simulink model "Open_scen_lucie_test_cs"  (R2019a)
settings: Solver=ode5  StartTime=0.0  StopTime=60  FixedStep=1/60  RelTol=1e-3
PreLoadFcn:
  | mbxruntime.callbacks.PreLoadFcn(bdroot);
PostLoadFcn:
  | mbxruntime.callbacks.PostLoadFcn(bdroot);
InitFcn:
  | mbxruntime.callbacks.InitFcn(bdroot);
StartFcn:
  | mbxruntime.callbacks.StartFcn(bdroot);
StopFcn:
  | mbxruntime.callbacks.StopFcn(bdroot);
model workspace: external: MAT-File .\Open_scen_lucie_test_cs_hws.mat (data not in the file)
undefined symbols (not defined in the file or in its folder): DiscIntNeverNeededParam, FovAzimuth, FovAzimuthDefined, FovElevation, FovElevationDefined, InitImageOutputDir, LocationX, LocationXDefined, LocationY, LocationYDefined, LocationZ, LocationZDefined, mbxruntime, Open_scen_lucie_test_cs_05b3fdca6ec99adc, Open_scen_lucie_test_cs_2d1bc0fbf6141b87, Open_scen_lucie_test_cs_453760b7ad36561d, Open_scen_lucie_test_cs_54de7300b247ce0d, Open_scen_lucie_test_cs_6819f386244a4b71, Open_scen_lucie_test_cs_685351e056f1bd0b, Open_scen_lucie_test_cs_6cd7f038842b0b77, Open_scen_lucie_test_cs_7a35ff65ce771bf6, Open_scen_lucie_test_cs_7ca083c9065fb1a1, Open_scen_lucie_test_cs_8bffacb258fa391b, Open_scen_lucie_test_cs_90e3bd399387ee5e, Open_scen_lucie_test_cs_a1176fb0c2e52fd1, Open_scen_lucie_test_cs_bb93306955583605, Open_scen_lucie_test_cs_c100ca66a180e443, Open_scen_lucie_test_cs_c1ddb1ec4c47a5f8, Open_scen_lucie_test_cs_ee3cfcef3d4d50fa, Open_scen_lucie_test_cs_f0142b471b498fb5, Open_scen_lucie_test_cs_fad1968c5de81336, OrientationPitch, OrientationPitchDefined, OrientationRoll, OrientationRollDefined, OrientationYaw, OrientationYawDefined, tabledata
libraries: adeye_lib x15, PreScanSimulinkLibrary x6, PreScanUsefulBlocks x1, simulink x1
(part 2 of 8)

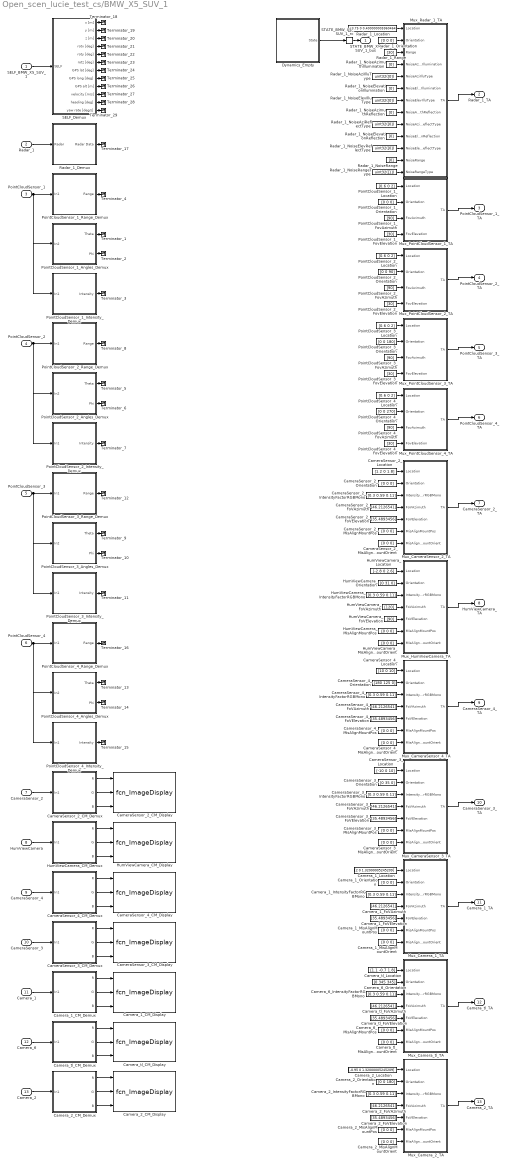
== system Open_scen_lucie_test_cs/BMW_X5_SUV_1 ==
  SELF_BMW_X5_SUV_1 : Inport  Tag=inport/SelfPort  OutDataTypeStr=Bus: PRESCAN_SELFSENSORDATA  PortDimensions=1  SampleTime=1/60  BusOutputAsStruct=on
  Radar_1 : Inport  Tag=inport/Radar  Port=2  OutDataTypeStr=Bus: PRESCAN_SCANNERSENSOR_MESSAGE  PortDimensions=7  SampleTime=1/20  BusOutputAsStruct=on
  PointCloudSensor_1 : Inport  Tag=inport/PointCloudInport  Port=3  OutDataTypeStr=single  SampleTime=1/20  BusOutputAsStruct=on
  PointCloudSensor_2 : Inport  Tag=inport/PointCloudInport  Port=4  OutDataTypeStr=single  SampleTime=1/20  BusOutputAsStruct=on
  PointCloudSensor_3 : Inport  Tag=inport/PointCloudInport  Port=5  OutDataTypeStr=single  SampleTime=1/20  BusOutputAsStruct=on
  PointCloudSensor_4 : Inport  Tag=inport/PointCloudInport  Port=6  OutDataTypeStr=single  SampleTime=1/20  BusOutputAsStruct=on
  CameraSensor_2 : Inport  Tag=inport/Camera/CameraSensor  Port=7  OutDataTypeStr=uint8  SampleTime=1/20  BusOutputAsStruct=on
  HumViewCamera : Inport  Tag=inport/Camera/CameraSensor  Port=8  OutDataTypeStr=uint8  SampleTime=1/60  BusOutputAsStruct=on
  CameraSensor_4 : Inport  Tag=inport/Camera/CameraSensor  Port=9  OutDataTypeStr=uint8  SampleTime=1/20  BusOutputAsStruct=on
  CameraSensor_3 : Inport  Tag=inport/Camera/CameraSensor  Port=10  OutDataTypeStr=uint8  SampleTime=1/20  BusOutputAsStruct=on
  Camera_1 : Inport  Tag=inport/Camera/CameraSensor  Port=11  OutDataTypeStr=uint8  SampleTime=1/20  BusOutputAsStruct=on
  Camera_tl : Inport  Tag=inport/Camera/CameraSensor  Port=12  OutDataTypeStr=uint8  SampleTime=1/20  BusOutputAsStruct=on
  Camera_2 : Inport  Tag=inport/Camera/CameraSensor  Port=13  OutDataTypeStr=uint8  SampleTime=1/20  BusOutputAsStruct=on
  CameraSensor_2_CM_Demux : Subsystem  Tag=demux/Camera/Color  mask{SensorName=CameraSensor_2, hres=960, vres=720}
      mask prompts: SensorName "Sensor Name"; hres "Horizontal Resolution"; vres "Vertical Resolution"
      mask Help: eval('openHelp(457)')
      mask Display:
      | fprintf('MONO CAMERA:\n Color\n %s \n %d x %d px',SensorName,hres,vres)
      | port_label('output',1,'R')
      | port_label('output',2,'G')
      | port_label('output',3,'B')
  CameraSensor_2_CM_Display : M-S-Function  Tag=CameraSensor_Color_Display  InitFcn=InitImageOutputDir(gcb);  FunctionName=fcn_ImageDisplay  Parameters=SensorName EnableDisplay EnablePosition DisplayPosition FigureHandle SaveResults BitmapFormat TempOutputDir CameraType DataType  mask(PreScan Color Display Block){SensorName=CameraSensor_2, EnableDisplay=on, EnablePosition=off, DisplayPosition=[10 10 960 720], FigureHandle=40605, SaveResults=off, Format=PNG, TempOutputDir=0, CameraType=Mono, DataType=uint8}
      mask prompts: SensorName "User Specified: Title of Display"; EnableDisplay "Active"; EnablePosition "Set Display window position"; DisplayPosition "Display window position [xpos ypos width height]"; FigureHandle "Unique Handle"; SaveResults "Save results"; TempOutputDir "OutputDir"; CameraType "Camera Type"; DataType "Image Data Type"
      mask help: This block displays the RGB output of a PreScan camera sensor.
      mask init:
      | if EnableDisplay
      |     EnableString='';
      |     EnableColor='gray';
      | else
      |     EnableString='INACTIVE';
      |     EnableColor='red';
      | end
      | switch Format
      |     case 1
      |         BitmapFormat = 'png';
      |     case 2
      |         BitmapFormat = 'bmp';
      |     case 3
      |         BitmapFormat = 'jpg';
      | end 
      | if CameraType==1
      |     CameraTypeName='MONO';
      |     PortNumber=0;
      | else
      |     CameraTypeName='STEREO';
      |     PortNumber=3;
      | end
      settings: CopyFcn=CopyFcnDisplay  DeleteFcn=PreScanBlockDeleteFcn;  ModelCloseFcn=fcn_ImageDisplay_ModelCloseFcn
      mask Help: eval('openHelp(457)')
      mask Callback EnablePosition:
      | MV=get_param(gcb,'MaskVisibilities');
      | if strcmp(get_param(gcb,'EnablePosition'),'on')
      |     MV{4}='on';
      | else
      |     MV{4}='off';
      | end
      | set_param(gcb,'MaskVisibilities',MV);
      | clear MV;
      mask TypeOptions Format: PNG | BMP | JPG
      mask TypeOptions CameraType: Mono | Stereo
      mask TypeOptions DataType: uint8 | single
      mask Display:
      | color(EnableColor);
      | fprintf('%s\n DISPLAY:\n Color \n %s',EnableString,SensorName)
      | port_label('input',1,'R')
      | port_label('input',2,'G')
      | port_label('input',3,'B')
      | port_label('input',PortNumber+1,'R')
      | port_label('input',PortNumber+2,'G')
      | port_label('input',PortNumber+3,'B')
  CameraSensor_2_FoVAzimuth : Constant  Tag=CameraSensor_2_FoVAzimuth  Value=[46.2126541]
  CameraSensor_2_FoVElevation : Constant  Tag=CameraSensor_2_FoVElevation  Value=[35.4893456]
  CameraSensor_2_IntensityFactorRGBMono : Constant  Tag=CameraSensor_2_IntensityFactorRGBMono  Value=[0.3 0.59 0.11]
  CameraSensor_2_Location : Constant  Tag=CameraSensor_2_Location  Value=[1.2 0 1.8]
  CameraSensor_2_MisAlignMountOrient : Constant  Tag=CameraSensor_2_MisAlignMountOrient  Value=[0 0 0]
  CameraSensor_2_MisAlignMountPos : Constant  Tag=CameraSensor_2_MisAlignMountPos  Value=[0 0 0]
  CameraSensor_2_Orientation : Constant  Tag=CameraSensor_2_Orientation  Value=[0 0 0]
  CameraSensor_3_CM_Demux : Subsystem  Tag=demux/Camera/Color  mask{SensorName=CameraSensor_3, hres=960, vres=720}
      mask prompts: SensorName "Sensor Name"; hres "Horizontal Resolution"; vres "Vertical Resolution"
      mask Help: eval('openHelp(457)')
      mask Display:
      | fprintf('MONO CAMERA:\n Color\n %s \n %d x %d px',SensorName,hres,vres)
      | port_label('output',1,'R')
      | port_label('output',2,'G')
      | port_label('output',3,'B')
  CameraSensor_3_CM_Display : M-S-Function  Tag=CameraSensor_Color_Display  InitFcn=InitImageOutputDir(gcb);  FunctionName=fcn_ImageDisplay  Parameters=SensorName EnableDisplay EnablePosition DisplayPosition FigureHandle SaveResults BitmapFormat TempOutputDir CameraType DataType  mask(PreScan Color Display Block){SensorName=CameraSensor_3, EnableDisplay=on, EnablePosition=off, DisplayPosition=[10 10 960 720], FigureHandle=40608, SaveResults=off, Format=PNG, TempOutputDir=0, CameraType=Mono, DataType=uint8}
      mask prompts: SensorName "User Specified: Title of Display"; EnableDisplay "Active"; EnablePosition "Set Display window position"; DisplayPosition "Display window position [xpos ypos width height]"; FigureHandle "Unique Handle"; SaveResults "Save results"; TempOutputDir "OutputDir"; CameraType "Camera Type"; DataType "Image Data Type"
      mask help: This block displays the RGB output of a PreScan camera sensor.
      mask init: same as Open_scen_lucie_test_cs/BMW_X5_SUV_1/CameraSensor_2_CM_Display
      settings: CopyFcn=CopyFcnDisplay  DeleteFcn=PreScanBlockDeleteFcn;  ModelCloseFcn=fcn_ImageDisplay_ModelCloseFcn
      mask Help: eval('openHelp(457)')
      mask Callback EnablePosition:
      | MV=get_param(gcb,'MaskVisibilities');
      | if strcmp(get_param(gcb,'EnablePosition'),'on')
      |     MV{4}='on';
      | else
      |     MV{4}='off';
      | end
      | set_param(gcb,'MaskVisibilities',MV);
      | clear MV;
      mask TypeOptions Format: PNG | BMP | JPG
      mask TypeOptions CameraType: Mono | Stereo
      mask TypeOptions DataType: uint8 | single
      mask Display:
      | color(EnableColor);
      | fprintf('%s\n DISPLAY:\n Color \n %s',EnableString,SensorName)
      | port_label('input',1,'R')
      | port_label('input',2,'G')
      | port_label('input',3,'B')
      | port_label('input',PortNumber+1,'R')
      | port_label('input',PortNumber+2,'G')
      | port_label('input',PortNumber+3,'B')
  CameraSensor_3_FoVAzimuth : Constant  Tag=CameraSensor_3_FoVAzimuth  Value=[46.2126541]
  CameraSensor_3_FoVElevation : Constant  Tag=CameraSensor_3_FoVElevation  Value=[35.4893456]
  CameraSensor_3_IntensityFactorRGBMono : Constant  Tag=CameraSensor_3_IntensityFactorRGBMono  Value=[0.3 0.59 0.11]
  CameraSensor_3_Location : Constant  Tag=CameraSensor_3_Location  Value=[-10 0 10]
  CameraSensor_3_MisAlignMountOrient : Constant  Tag=CameraSensor_3_MisAlignMountOrient  Value=[0 0 0]
  CameraSensor_3_MisAlignMountPos : Constant  Tag=CameraSensor_3_MisAlignMountPos  Value=[0 0 0]
  CameraSensor_3_Orientation : Constant  Tag=CameraSensor_3_Orientation  Value=[0 35 0]
  CameraSensor_4_CM_Demux : Subsystem  Tag=demux/Camera/Color  mask{SensorName=CameraSensor_4, hres=960, vres=720}
      mask prompts: SensorName "Sensor Name"; hres "Horizontal Resolution"; vres "Vertical Resolution"
      mask Help: eval('openHelp(457)')
      mask Display:
      | fprintf('MONO CAMERA:\n Color\n %s \n %d x %d px',SensorName,hres,vres)
      | port_label('output',1,'R')
      | port_label('output',2,'G')
      | port_label('output',3,'B')
  CameraSensor_4_CM_Display : M-S-Function  Tag=CameraSensor_Color_Display  InitFcn=InitImageOutputDir(gcb);  FunctionName=fcn_ImageDisplay  Parameters=SensorName EnableDisplay EnablePosition DisplayPosition FigureHandle SaveResults BitmapFormat TempOutputDir CameraType DataType  mask(PreScan Color Display Block){SensorName=CameraSensor_4, EnableDisplay=on, EnablePosition=off, DisplayPosition=[10 10 960 720], FigureHandle=40607, SaveResults=off, Format=PNG, TempOutputDir=0, CameraType=Mono, DataType=uint8}
      mask prompts: SensorName "User Specified: Title of Display"; EnableDisplay "Active"; EnablePosition "Set Display window position"; DisplayPosition "Display window position [xpos ypos width height]"; FigureHandle "Unique Handle"; SaveResults "Save results"; TempOutputDir "OutputDir"; CameraType "Camera Type"; DataType "Image Data Type"
      mask help: This block displays the RGB output of a PreScan camera sensor.
      mask init: same as Open_scen_lucie_test_cs/BMW_X5_SUV_1/CameraSensor_2_CM_Display
      settings: CopyFcn=CopyFcnDisplay  DeleteFcn=PreScanBlockDeleteFcn;  ModelCloseFcn=fcn_ImageDisplay_ModelCloseFcn
      mask Help: eval('openHelp(457)')
      mask Callback EnablePosition:
      | MV=get_param(gcb,'MaskVisibilities');
      | if strcmp(get_param(gcb,'EnablePosition'),'on')
      |     MV{4}='on';
      | else
      |     MV{4}='off';
      | end
      | set_param(gcb,'MaskVisibilities',MV);
      | clear MV;
      mask TypeOptions Format: PNG | BMP | JPG
      mask TypeOptions CameraType: Mono | Stereo
      mask TypeOptions DataType: uint8 | single
      mask Display:
      | color(EnableColor);
      | fprintf('%s\n DISPLAY:\n Color \n %s',EnableString,SensorName)
      | port_label('input',1,'R')
      | port_label('input',2,'G')
      | port_label('input',3,'B')
      | port_label('input',PortNumber+1,'R')
      | port_label('input',PortNumber+2,'G')
      | port_label('input',PortNumber+3,'B')
  CameraSensor_4_FoVAzimuth : Constant  Tag=CameraSensor_4_FoVAzimuth  Value=[46.2126541]
  CameraSensor_4_FoVElevation : Constant  Tag=CameraSensor_4_FoVElevation  Value=[35.4893456]
  CameraSensor_4_IntensityFactorRGBMono : Constant  Tag=CameraSensor_4_IntensityFactorRGBMono  Value=[0.3 0.59 0.11]
  CameraSensor_4_Location : Constant  Tag=CameraSensor_4_Location  Value=[10 0 10]
  CameraSensor_4_MisAlignMountOrient : Constant  Tag=CameraSensor_4_MisAlignMountOrient  Value=[0 0 0]
  CameraSensor_4_MisAlignMountPos : Constant  Tag=CameraSensor_4_MisAlignMountPos  Value=[0 0 0]
  CameraSensor_4_Orientation : Constant  Tag=CameraSensor_4_Orientation  Value=[180 125 0]
  Camera_1_CM_Demux : Subsystem  Tag=demux/Camera/Color  mask{SensorName=Camera_1, hres=960, vres=720}
      mask prompts: SensorName "Sensor Name"; hres "Horizontal Resolution"; vres "Vertical Resolution"
      mask Help: eval('openHelp(457)')
      mask Display:
      | fprintf('MONO CAMERA:\n Color\n %s \n %d x %d px',SensorName,hres,vres)
      | port_label('output',1,'R')
      | port_label('output',2,'G')
      | port_label('output',3,'B')
  Camera_1_CM_Display : M-S-Function  Tag=CameraSensor_Color_Display  InitFcn=InitImageOutputDir(gcb);  FunctionName=fcn_ImageDisplay  Parameters=SensorName EnableDisplay EnablePosition DisplayPosition FigureHandle SaveResults BitmapFormat TempOutputDir CameraType DataType  mask(PreScan Color Display Block){SensorName=Camera_1, EnableDisplay=on, EnablePosition=off, DisplayPosition=[10 10 960 720], FigureHandle=40609, SaveResults=off, Format=PNG, TempOutputDir=0, CameraType=Mono, DataType=uint8}
      mask prompts: SensorName "User Specified: Title of Display"; EnableDisplay "Active"; EnablePosition "Set Display window position"; DisplayPosition "Display window position [xpos ypos width height]"; FigureHandle "Unique Handle"; SaveResults "Save results"; TempOutputDir "OutputDir"; CameraType "Camera Type"; DataType "Image Data Type"
      mask help: This block displays the RGB output of a PreScan camera sensor.
      mask init: same as Open_scen_lucie_test_cs/BMW_X5_SUV_1/CameraSensor_2_CM_Display
      settings: CopyFcn=CopyFcnDisplay  DeleteFcn=PreScanBlockDeleteFcn;  ModelCloseFcn=fcn_ImageDisplay_ModelCloseFcn
      mask Help: eval('openHelp(457)')
      mask Callback EnablePosition:
      | MV=get_param(gcb,'MaskVisibilities');
      | if strcmp(get_param(gcb,'EnablePosition'),'on')
      |     MV{4}='on';
      | else
      |     MV{4}='off';
      | end
      | set_param(gcb,'MaskVisibilities',MV);
      | clear MV;
      mask TypeOptions Format: PNG | BMP | JPG
      mask TypeOptions CameraType: Mono | Stereo
      mask TypeOptions DataType: uint8 | single
      mask Display:
      | color(EnableColor);
      | fprintf('%s\n DISPLAY:\n Color \n %s',EnableString,SensorName)
      | port_label('input',1,'R')
      | port_label('input',2,'G')
      | port_label('input',3,'B')
      | port_label('input',PortNumber+1,'R')
      | port_label('input',PortNumber+2,'G')
      | port_label('input',PortNumber+3,'B')
  Camera_1_FoVAzimuth : Constant  Tag=Camera_1_FoVAzimuth  Value=[46.2126541]
  Camera_1_FoVElevation : Constant  Tag=Camera_1_FoVElevation  Value=[35.4893456]
  Camera_1_IntensityFactorRGBMono : Constant  Tag=Camera_1_IntensityFactorRGBMono  Value=[0.3 0.59 0.11]
  Camera_1_Location : Constant  Tag=Camera_1_Location  Value=[2 0 1.32000005245209]
  Camera_1_MisAlignMountOrient : Constant  Tag=Camera_1_MisAlignMountOrient  Value=[0 0 0]
  Camera_1_MisAlignMountPos : Constant  Tag=Camera_1_MisAlignMountPos  Value=[0 0 0]
  Camera_1_Orientation : Constant  Tag=Camera_1_Orientation  Value=[0 0 0]
  Camera_2_CM_Demux : Subsystem  Tag=demux/Camera/Color  mask{SensorName=Camera_2, hres=960, vres=720}
      mask prompts: SensorName "Sensor Name"; hres "Horizontal Resolution"; vres "Vertical Resolution"
      mask Help: eval('openHelp(457)')
      mask Display:
      | fprintf('MONO CAMERA:\n Color\n %s \n %d x %d px',SensorName,hres,vres)
      | port_label('output',1,'R')
      | port_label('output',2,'G')
      | port_label('output',3,'B')
  Camera_2_CM_Display : M-S-Function  Tag=CameraSensor_Color_Display  InitFcn=InitImageOutputDir(gcb);  FunctionName=fcn_ImageDisplay  Parameters=SensorName EnableDisplay EnablePosition DisplayPosition FigureHandle SaveResults BitmapFormat TempOutputDir CameraType DataType  mask(PreScan Color Display Block){SensorName=Camera_2, EnableDisplay=on, EnablePosition=off, DisplayPosition=[10 10 960 720], FigureHandle=40611, SaveResults=off, Format=PNG, TempOutputDir=0, CameraType=Mono, DataType=uint8}
      mask prompts: SensorName "User Specified: Title of Display"; EnableDisplay "Active"; EnablePosition "Set Display window position"; DisplayPosition "Display window position [xpos ypos width height]"; FigureHandle "Unique Handle"; SaveResults "Save results"; TempOutputDir "OutputDir"; CameraType "Camera Type"; DataType "Image Data Type"
      mask help: This block displays the RGB output of a PreScan camera sensor.
      mask init: same as Open_scen_lucie_test_cs/BMW_X5_SUV_1/CameraSensor_2_CM_Display
      settings: CopyFcn=CopyFcnDisplay  DeleteFcn=PreScanBlockDeleteFcn;  ModelCloseFcn=fcn_ImageDisplay_ModelCloseFcn
      mask Help: eval('openHelp(457)')
      mask Callback EnablePosition:
      | MV=get_param(gcb,'MaskVisibilities');
      | if strcmp(get_param(gcb,'EnablePosition'),'on')
      |     MV{4}='on';
      | else
      |     MV{4}='off';
      | end
      | set_param(gcb,'MaskVisibilities',MV);
      | clear MV;
      mask TypeOptions Format: PNG | BMP | JPG
      mask TypeOptions CameraType: Mono | Stereo
      mask TypeOptions DataType: uint8 | single
      mask Display:
      | color(EnableColor);
      | fprintf('%s\n DISPLAY:\n Color \n %s',EnableString,SensorName)
      | port_label('input',1,'R')
      | port_label('input',2,'G')
      | port_label('input',3,'B')
      | port_label('input',PortNumber+1,'R')
      | port_label('input',PortNumber+2,'G')
      | port_label('input',PortNumber+3,'B')
  Camera_2_FoVAzimuth : Constant  Tag=Camera_2_FoVAzimuth  Value=[46.2126541]
  Camera_2_FoVElevation : Constant  Tag=Camera_2_FoVElevation  Value=[35.4893456]
  Camera_2_IntensityFactorRGBMono : Constant  Tag=Camera_2_IntensityFactorRGBMono  Value=[0.3 0.59 0.11]
  Camera_2_Location : Constant  Tag=Camera_2_Location  Value=[-0.95 0 1.32000005245209]
  Camera_2_MisAlignMountOrient : Constant  Tag=Camera_2_MisAlignMountOrient  Value=[0 0 0]
  Camera_2_MisAlignMountPos : Constant  Tag=Camera_2_MisAlignMountPos  Value=[0 0 0]
  Camera_2_Orientation : Constant  Tag=Camera_2_Orientation  Value=[0 0 180]
  Camera_tl_CM_Demux : Subsystem  Tag=demux/Camera/Color  mask{SensorName=Camera_tl, hres=960, vres=720}
      mask prompts: SensorName "Sensor Name"; hres "Horizontal Resolution"; vres "Vertical Resolution"
      mask Help: eval('openHelp(457)')
      mask Display:
      | fprintf('MONO CAMERA:\n Color\n %s \n %d x %d px',SensorName,hres,vres)
      | port_label('output',1,'R')
      | port_label('output',2,'G')
      | port_label('output',3,'B')
  Camera_tl_CM_Display : M-S-Function  Tag=CameraSensor_Color_Display  InitFcn=InitImageOutputDir(gcb);  FunctionName=fcn_ImageDisplay  Parameters=SensorName EnableDisplay EnablePosition DisplayPosition FigureHandle SaveResults BitmapFormat TempOutputDir CameraType DataType  mask(PreScan Color Display Block){SensorName=Camera_tl, EnableDisplay=on, EnablePosition=off, DisplayPosition=[10 10 960 720], FigureHandle=40610, SaveResults=off, Format=PNG, TempOutputDir=0, CameraType=Mono, DataType=uint8}
      mask prompts: SensorName "User Specified: Title of Display"; EnableDisplay "Active"; EnablePosition "Set Display window position"; DisplayPosition "Display window position [xpos ypos width height]"; FigureHandle "Unique Handle"; SaveResults "Save results"; TempOutputDir "OutputDir"; CameraType "Camera Type"; DataType "Image Data Type"
      mask help: This block displays the RGB output of a PreScan camera sensor.
      mask init: same as Open_scen_lucie_test_cs/BMW_X5_SUV_1/CameraSensor_2_CM_Display
      settings: CopyFcn=CopyFcnDisplay  DeleteFcn=PreScanBlockDeleteFcn;  ModelCloseFcn=fcn_ImageDisplay_ModelCloseFcn
      mask Help: eval('openHelp(457)')
      mask Callback EnablePosition:
      | MV=get_param(gcb,'MaskVisibilities');
      | if strcmp(get_param(gcb,'EnablePosition'),'on')
      |     MV{4}='on';
      | else
      |     MV{4}='off';
      | end
      | set_param(gcb,'MaskVisibilities',MV);
      | clear MV;
      mask TypeOptions Format: PNG | BMP | JPG
      mask TypeOptions CameraType: Mono | Stereo
      mask TypeOptions DataType: uint8 | single
      mask Display:
      | color(EnableColor);
      | fprintf('%s\n DISPLAY:\n Color \n %s',EnableString,SensorName)
      | port_label('input',1,'R')
      | port_label('input',2,'G')
      | port_label('input',3,'B')
      | port_label('input',PortNumber+1,'R')
      | port_label('input',PortNumber+2,'G')
      | port_label('input',PortNumber+3,'B')
  Camera_tl_FoVAzimuth : Constant  Tag=Camera_tl_FoVAzimuth  Value=[46.2126541]
  Camera_tl_FoVElevation : Constant  Tag=Camera_tl_FoVElevation  Value=[35.4893456]
  Camera_tl_IntensityFactorRGBMono : Constant  Tag=Camera_tl_IntensityFactorRGBMono  Value=[0.3 0.59 0.11]
  Camera_tl_Location : Constant  Tag=Camera_tl_Location  Value=[1.1 -0.7 1.8]
  Camera_tl_MisAlignMountOrient : Constant  Tag=Camera_tl_MisAlignMountOrient  Value=[0 0 0]
  Camera_tl_MisAlignMountPos : Constant  Tag=Camera_tl_MisAlignMountPos  Value=[0 0 0]
  Camera_tl_Orientation : Constant  Tag=Camera_tl_Orientation  Value=[0 345 345]
  Dynamics_Empty : Subsystem  Tag=Dynamics_Empty
      mask Help: eval('openHelp(202)')
      mask Display: port_label('output', 1, 'State');text(0,0,' Empty\n')
  HumViewCamera_CM_Demux : Subsystem  Tag=demux/Camera/Color  mask{SensorName=HumViewCamera, hres=1871, vres=1080}
      mask prompts: SensorName "Sensor Name"; hres "Horizontal Resolution"; vres "Vertical Resolution"
      mask Help: eval('openHelp(457)')
      mask Display:
      | fprintf('MONO CAMERA:\n Color\n %s \n %d x %d px',SensorName,hres,vres)
      | port_label('output',1,'R')
      | port_label('output',2,'G')
      | port_label('output',3,'B')
  HumViewCamera_CM_Display : M-S-Function  Tag=CameraSensor_Color_Display  InitFcn=InitImageOutputDir(gcb);  FunctionName=fcn_ImageDisplay  Parameters=SensorName EnableDisplay EnablePosition DisplayPosition FigureHandle SaveResults BitmapFormat TempOutputDir CameraType DataType  mask(PreScan Color Display Block){SensorName=HumViewCamera, EnableDisplay=on, EnablePosition=off, DisplayPosition=[10 10 1871 1080], FigureHandle=40606, SaveResults=off, Format=PNG, TempOutputDir=0, CameraType=Mono, DataType=uint8}
      mask prompts: SensorName "User Specified: Title of Display"; EnableDisplay "Active"; EnablePosition "Set Display window position"; DisplayPosition "Display window position [xpos ypos width height]"; FigureHandle "Unique Handle"; SaveResults "Save results"; TempOutputDir "OutputDir"; CameraType "Camera Type"; DataType "Image Data Type"
      mask help: This block displays the RGB output of a PreScan camera sensor.
      mask init: same as Open_scen_lucie_test_cs/BMW_X5_SUV_1/CameraSensor_2_CM_Display
      settings: CopyFcn=CopyFcnDisplay  DeleteFcn=PreScanBlockDeleteFcn;  ModelCloseFcn=fcn_ImageDisplay_ModelCloseFcn
      mask Help: eval('openHelp(457)')
      mask Callback EnablePosition:
      | MV=get_param(gcb,'MaskVisibilities');
      | if strcmp(get_param(gcb,'EnablePosition'),'on')
      |     MV{4}='on';
      | else
      |     MV{4}='off';
      | end
      | set_param(gcb,'MaskVisibilities',MV);
      | clear MV;
      mask TypeOptions Format: PNG | BMP | JPG
      mask TypeOptions CameraType: Mono | Stereo
      mask TypeOptions DataType: uint8 | single
      mask Display:
      | color(EnableColor);
      | fprintf('%s\n DISPLAY:\n Color \n %s',EnableString,SensorName)
      | port_label('input',1,'R')
      | port_label('input',2,'G')
      | port_label('input',3,'B')
      | port_label('input',PortNumber+1,'R')
      | port_label('input',PortNumber+2,'G')
      | port_label('input',PortNumber+3,'B')
  HumViewCamera_FoVAzimuth : Constant  Tag=HumViewCamera_FoVAzimuth  Value=[120]
  HumViewCamera_FoVElevation : Constant  Tag=HumViewCamera_FoVElevation  Value=[90]
  HumViewCamera_IntensityFactorRGBMono : Constant  Tag=HumViewCamera_IntensityFactorRGBMono  Value=[0.3 0.59 0.11]
  HumViewCamera_Location : Constant  Tag=HumViewCamera_Location  Value=[-2.8 0 2.6]
  HumViewCamera_MisAlignMountOrient : Constant  Tag=HumViewCamera_MisAlignMountOrient  Value=[0 0 0]
  HumViewCamera_MisAlignMountPos : Constant  Tag=HumViewCamera_MisAlignMountPos  Value=[0 0 0]
  HumViewCamera_Orientation : Constant  Tag=HumViewCamera_Orientation  Value=[0 31 0]
  Mux_CameraSensor_2_TA : Subsystem  Tag=mux/Camera_TA/CameraSensor
  Mux_CameraSensor_3_TA : Subsystem  Tag=mux/Camera_TA/CameraSensor
  Mux_CameraSensor_4_TA : Subsystem  Tag=mux/Camera_TA/CameraSensor
  Mux_Camera_1_TA : Subsystem  Tag=mux/Camera_TA/CameraSensor
  Mux_Camera_2_TA : Subsystem  Tag=mux/Camera_TA/CameraSensor
  Mux_Camera_tl_TA : Subsystem  Tag=mux/Camera_TA/CameraSensor
  Mux_HumViewCamera_TA : Subsystem  Tag=mux/Camera_TA/CameraSensor
  Mux_PointCloudSensor_1_TA : Subsystem  Tag=mux/SensorTA
  Mux_PointCloudSensor_2_TA : Subsystem  Tag=mux/SensorTA
  Mux_PointCloudSensor_3_TA : Subsystem  Tag=mux/SensorTA
  Mux_PointCloudSensor_4_TA : Subsystem  Tag=mux/SensorTA
  Mux_Radar_1_TA : Subsystem  Tag=mux/Radar_TA
  PointCloudSensor_1_Angles_Demux : Subsystem  Tag=demux/PCS/Angles  mask{SensorName=PointCloudSensor_1, offset=225, hres=225, vres=16}
      mask prompts: SensorName "Sensor Name"; offset "Data Start"; hres "Horizontal Resolution"; vres "Vertical Resolution"
      mask Help: eval('openHelp(6400)')
      mask Display:
      | fprintf('Point Cloud:\n Data\n %s \n %d x %d px',SensorName,hres,vres)
      | port_label('output',1,'Theta')
      | port_label('output',2,'Phi')
  PointCloudSensor_1_FovAzimuth : Constant  Tag=PointCloudSensor_1_FovAzimuth  Value=[90]
  PointCloudSensor_1_FovElevation : Constant  Tag=PointCloudSensor_1_FovElevation  Value=[30]
  PointCloudSensor_1_Intensity_Demux : Subsystem  Tag=demux/PCS/Intensity  mask{SensorName=PointCloudSensor_1, offset=675, hres=225, vres=16}
      mask prompts: SensorName "Sensor Name"; offset "Data Start"; hres "Horizontal Resolution"; vres "Vertical Resolution"
      mask Help: eval('openHelp(6400)')
      mask Display:
      | fprintf('Point Cloud:\n Data\n %s \n %d x %d px',SensorName,hres,vres)
      | port_label('output',1,'Intensity')
  PointCloudSensor_1_Location : Constant  Tag=PointCloudSensor_1_Location  Value=[0.6 0 2]
  PointCloudSensor_1_Orientation : Constant  Tag=PointCloudSensor_1_Orientation  Value=[0 0 0]
  PointCloudSensor_1_Range_Demux : Subsystem  Tag=demux/PCS/Range  mask{SensorName=PointCloudSensor_1, offset=0, hres=225, vres=16}
      mask prompts: SensorName "Sensor Name"; offset "Data Start"; hres "Horizontal Resolution"; vres "Vertical Resolution"
      mask Help: eval('openHelp(6400)')
      mask Display:
      | fprintf('Point Cloud:\n Data\n %s \n %d x %d px',SensorName,hres,vres)
      | port_label('output',1,'Range')
  PointCloudSensor_2_Angles_Demux : Subsystem  Tag=demux/PCS/Angles  mask{SensorName=PointCloudSensor_2, offset=225, hres=225, vres=16}
      mask prompts: SensorName "Sensor Name"; offset "Data Start"; hres "Horizontal Resolution"; vres "Vertical Resolution"
      mask Help: eval('openHelp(6400)')
      mask Display:
      | fprintf('Point Cloud:\n Data\n %s \n %d x %d px',SensorName,hres,vres)
      | port_label('output',1,'Theta')
      | port_label('output',2,'Phi')
  PointCloudSensor_2_FovAzimuth : Constant  Tag=PointCloudSensor_2_FovAzimuth  Value=[90]
  PointCloudSensor_2_FovElevation : Constant  Tag=PointCloudSensor_2_FovElevation  Value=[30]
  PointCloudSensor_2_Intensity_Demux : Subsystem  Tag=demux/PCS/Intensity  mask{SensorName=PointCloudSensor_2, offset=675, hres=225, vres=16}
      mask prompts: SensorName "Sensor Name"; offset "Data Start"; hres "Horizontal Resolution"; vres "Vertical Resolution"
      mask Help: eval('openHelp(6400)')
      mask Display:
      | fprintf('Point Cloud:\n Data\n %s \n %d x %d px',SensorName,hres,vres)
      | port_label('output',1,'Intensity')
  PointCloudSensor_2_Location : Constant  Tag=PointCloudSensor_2_Location  Value=[0.6 0 2]
  PointCloudSensor_2_Orientation : Constant  Tag=PointCloudSensor_2_Orientation  Value=[0 0 90]
  PointCloudSensor_2_Range_Demux : Subsystem  Tag=demux/PCS/Range  mask{SensorName=PointCloudSensor_2, offset=0, hres=225, vres=16}
      mask prompts: SensorName "Sensor Name"; offset "Data Start"; hres "Horizontal Resolution"; vres "Vertical Resolution"
      mask Help: eval('openHelp(6400)')
      mask Display:
      | fprintf('Point Cloud:\n Data\n %s \n %d x %d px',SensorName,hres,vres)
      | port_label('output',1,'Range')
  PointCloudSensor_3_Angles_Demux : Subsystem  Tag=demux/PCS/Angles  mask{SensorName=PointCloudSensor_3, offset=225, hres=225, vres=16}
      mask prompts: SensorName "Sensor Name"; offset "Data Start"; hres "Horizontal Resolution"; vres "Vertical Resolution"
      mask Help: eval('openHelp(6400)')
      mask Display:
      | fprintf('Point Cloud:\n Data\n %s \n %d x %d px',SensorName,hres,vres)
      | port_label('output',1,'Theta')
      | port_label('output',2,'Phi')
  PointCloudSensor_3_FovAzimuth : Constant  Tag=PointCloudSensor_3_FovAzimuth  Value=[90]
  PointCloudSensor_3_FovElevation : Constant  Tag=PointCloudSensor_3_FovElevation  Value=[30]
  PointCloudSensor_3_Intensity_Demux : Subsystem  Tag=demux/PCS/Intensity  mask{SensorName=PointCloudSensor_3, offset=675, hres=225, vres=16}
      mask prompts: SensorName "Sensor Name"; offset "Data Start"; hres "Horizontal Resolution"; vres "Vertical Resolution"
      mask Help: eval('openHelp(6400)')
      mask Display:
      | fprintf('Point Cloud:\n Data\n %s \n %d x %d px',SensorName,hres,vres)
      | port_label('output',1,'Intensity')
  PointCloudSensor_3_Location : Constant  Tag=PointCloudSensor_3_Location  Value=[0.6 0 2]
  PointCloudSensor_3_Orientation : Constant  Tag=PointCloudSensor_3_Orientation  Value=[0 0 180]
  PointCloudSensor_3_Range_Demux : Subsystem  Tag=demux/PCS/Range  mask{SensorName=PointCloudSensor_3, offset=0, hres=225, vres=16}
      mask prompts: SensorName "Sensor Name"; offset "Data Start"; hres "Horizontal Resolution"; vres "Vertical Resolution"
      mask Help: eval('openHelp(6400)')
      mask Display:
      | fprintf('Point Cloud:\n Data\n %s \n %d x %d px',SensorName,hres,vres)
      | port_label('output',1,'Range')
  PointCloudSensor_4_Angles_Demux : Subsystem  Tag=demux/PCS/Angles  mask{SensorName=PointCloudSensor_4, offset=225, hres=225, vres=16}
      mask prompts: SensorName "Sensor Name"; offset "Data Start"; hres "Horizontal Resolution"; vres "Vertical Resolution"
      mask Help: eval('openHelp(6400)')
      mask Display:
      | fprintf('Point Cloud:\n Data\n %s \n %d x %d px',SensorName,hres,vres)
      | port_label('output',1,'Theta')
      | port_label('output',2,'Phi')
  PointCloudSensor_4_FovAzimuth : Constant  Tag=PointCloudSensor_4_FovAzimuth  Value=[90]
  PointCloudSensor_4_FovElevation : Constant  Tag=PointCloudSensor_4_FovElevation  Value=[30]
  PointCloudSensor_4_Intensity_Demux : Subsystem  Tag=demux/PCS/Intensity  mask{SensorName=PointCloudSensor_4, offset=675, hres=225, vres=16}
      mask prompts: SensorName "Sensor Name"; offset "Data Start"; hres "Horizontal Resolution"; vres "Vertical Resolution"
      mask Help: eval('openHelp(6400)')
      mask Display:
      | fprintf('Point Cloud:\n Data\n %s \n %d x %d px',SensorName,hres,vres)
      | port_label('output',1,'Intensity')
  PointCloudSensor_4_Location : Constant  Tag=PointCloudSensor_4_Location  Value=[0.6 0 2]
  PointCloudSensor_4_Orientation : Constant  Tag=PointCloudSensor_4_Orientation  Value=[0 0 270]
  PointCloudSensor_4_Range_Demux : Subsystem  Tag=demux/PCS/Range  mask{SensorName=PointCloudSensor_4, offset=0, hres=225, vres=16}
      mask prompts: SensorName "Sensor Name"; offset "Data Start"; hres "Horizontal Resolution"; vres "Vertical Resolution"
      mask Help: eval('openHelp(6400)')
      mask Display:
      | fprintf('Point Cloud:\n Data\n %s \n %d x %d px',SensorName,hres,vres)
      | port_label('output',1,'Range')
  Radar_1_Demux : Subsystem  Tag=demux/Radar  TreatAsAtomicUnit=on  mask(PreScan Demux Block: Radar){MAXMESSAGES=7}
      mask prompts: MAXMESSAGES "Number of Objects"
      mask help:
      | The Radar Sensor is a detailed sensor based on a physical radar
      | model that includes Antenna GAIN Maps (AGM) and atmospheric
      | attenuation.
      |
      | For more information, please click Help.
      mask Help: eval('openHelp(1464)')
      mask Display:
      | port_label('input',1,'Radar')
      | port_label('output',1,'Radar Data')
  Radar_1_Location : Constant  Tag=Radar_1_Location  Value=[3.75 0 0.400000005960464]
  Radar_1_NoiseAziIlluType : Constant  Tag=Radar_1_NoiseAziIlluType  Value=uint32([0])
  Radar_1_NoiseAziReflectType : Constant  Tag=Radar_1_NoiseAziReflectType  Value=uint32([0])
  Radar_1_NoiseAzimuthIllumination : Constant  Tag=Radar_1_NoiseAzimuthIllumination  Value=[0]
  Radar_1_NoiseAzimuthReflection : Constant  Tag=Radar_1_NoiseAzimuthReflection  Value=[0]
  Radar_1_NoiseElevIlluType : Constant  Tag=Radar_1_NoiseElevIlluType  Value=uint32([0])
  Radar_1_NoiseElevReflectType : Constant  Tag=Radar_1_NoiseElevReflectType  Value=uint32([0])
  Radar_1_NoiseElevationIllumination : Constant  Tag=Radar_1_NoiseElevationIllumination  Value=[0]
  Radar_1_NoiseElevationReflection : Constant  Tag=Radar_1_NoiseElevationReflection  Value=[0]
  Radar_1_NoiseRange : Constant  Tag=Radar_1_NoiseRange  Value=[0]
  Radar_1_NoiseRangeType : Constant  Tag=Radar_1_NoiseRangeType  Value=uint32([1])
  Radar_1_Orientation : Constant  Tag=Radar_1_Orientation  Value=[0 0 0]
  Radar_1_Range : Constant  Tag=Radar_1_Range  Value=[30]
  SELF_Demux : Subsystem  Tag=demux/SelfPort  mask(PreScan Demux Block:){}
      mask help:
      | The SELF port shows (state) information of the actor itself. The outputs are position in the experiment's axis system and the GPS coordinates, and the object's absolute velocity and compass heading.
      |
      | For more information, please click Help.
      settings: DeleteFcn=PreScanBlockDeleteFcn;
      mask Help: eval('openHelp(462)')
      mask Display:
      | port_label('output',1,'x [m]')
      | port_label('output',2,'y [m]')
      | port_label('output',3,'z [m]','texmode','on')
      | port_label('output',4,'Rotx [deg]','texmode','on')
      | port_label('output',5,'Roty [deg]','texmode','on')
      | port_label('output',6,'Rotz [deg]','texmode','on')
      | port_label('output',7,'GPS lat [deg]','texmode','on')
      | port_label('output',8,'GPS long [deg]','texmode','on')
      | port_label('output',9,'GPS alt [m]','texmode','on')
      | port_label('output',10,'Velocity [m/s]')
      | port_label('output',11,'Heading [deg]')
      | port_label('output',12,'Yaw rate [deg/s]')
  STATE_BMW_X5_SUV_1_rc : RateTransition  Tag=mux_rc/StatePort  OutPortSampleTimeOpt=Inherit
  Terminator_{1..29} (29 alike) : Terminator
  STATE_BMW_X5_SUV_1_bus : Outport  Tag=outport/StatePort  OutDataTypeStr=Bus: PRESCAN_STATEACTUATORDATA  PortDimensions=1  SampleTime=1/60
  Radar_1_TA : Outport  Tag=outport/Radar_TA  Port=2  OutDataTypeStr=Bus: PRESCAN_SCANNERSENSOR_TA  PortDimensions=1  SampleTime=1/60
  PointCloudSensor_1_TA : Outport  Tag=outport/SensorTA  Port=3  OutDataTypeStr=Bus: PRESCAN_PCS_TA_DATA  PortDimensions=1  SampleTime=1/60
  PointCloudSensor_2_TA : Outport  Tag=outport/SensorTA  Port=4  OutDataTypeStr=Bus: PRESCAN_PCS_TA_DATA  PortDimensions=1  SampleTime=1/60
  PointCloudSensor_3_TA : Outport  Tag=outport/SensorTA  Port=5  OutDataTypeStr=Bus: PRESCAN_PCS_TA_DATA  PortDimensions=1  SampleTime=1/60
  PointCloudSensor_4_TA : Outport  Tag=outport/SensorTA  Port=6  OutDataTypeStr=Bus: PRESCAN_PCS_TA_DATA  PortDimensions=1  SampleTime=1/60
  CameraSensor_2_TA : Outport  Tag=outport/Camera_TA/CameraSensor  Port=7  OutDataTypeStr=Bus: PRESCAN_CAMERASENSOR_TA  PortDimensions=1  SampleTime=1/60
  HumViewCamera_TA : Outport  Tag=outport/Camera_TA/CameraSensor  Port=8  OutDataTypeStr=Bus: PRESCAN_CAMERASENSOR_TA  PortDimensions=1  SampleTime=1/60
  CameraSensor_4_TA : Outport  Tag=outport/Camera_TA/CameraSensor  Port=9  OutDataTypeStr=Bus: PRESCAN_CAMERASENSOR_TA  PortDimensions=1  SampleTime=1/60
  CameraSensor_3_TA : Outport  Tag=outport/Camera_TA/CameraSensor  Port=10  OutDataTypeStr=Bus: PRESCAN_CAMERASENSOR_TA  PortDimensions=1  SampleTime=1/60
  Camera_1_TA : Outport  Tag=outport/Camera_TA/CameraSensor  Port=11  OutDataTypeStr=Bus: PRESCAN_CAMERASENSOR_TA  PortDimensions=1  SampleTime=1/60
  Camera_tl_TA : Outport  Tag=outport/Camera_TA/CameraSensor  Port=12  OutDataTypeStr=Bus: PRESCAN_CAMERASENSOR_TA  PortDimensions=1  SampleTime=1/60
  Camera_2_TA : Outport  Tag=outport/Camera_TA/CameraSensor  Port=13  OutDataTypeStr=Bus: PRESCAN_CAMERASENSOR_TA  PortDimensions=1  SampleTime=1/60
  wires:
  STATE_BMW_X5_SUV_1_rc/1 -> STATE_BMW_X5_SUV_1_bus/1
  SELF_BMW_X5_SUV_1/1 -> SELF_Demux/1(SELF)
  Radar_1/1 -> Radar_1_Demux/1(Radar)
  Radar_1_Location/1 -> Mux_Radar_1_TA/1(Location)
  Radar_1_Orientation/1 -> Mux_Radar_1_TA/2(Orientation)
  Radar_1_Range/1 -> Mux_Radar_1_TA/3(Range)
  Radar_1_NoiseAzimuthIllumination/1 -> Mux_Radar_1_TA/4(NoiseAzimuthIllumination)
  Radar_1_NoiseAziIlluType/1 -> Mux_Radar_1_TA/5(NoiseAziIlluType)
  Radar_1_NoiseElevationIllumination/1 -> Mux_Radar_1_TA/6(NoiseElevationIllumination)
  Radar_1_NoiseElevIlluType/1 -> Mux_Radar_1_TA/7(NoiseElevIlluType)
  Radar_1_NoiseAzimuthReflection/1 -> Mux_Radar_1_TA/8(NoiseAzimuthReflection)
  Radar_1_NoiseAziReflectType/1 -> Mux_Radar_1_TA/9(NoiseAziReflectType)
  Radar_1_NoiseElevationReflection/1 -> Mux_Radar_1_TA/10(NoiseElevationReflection)
  Radar_1_NoiseElevReflectType/1 -> Mux_Radar_1_TA/11(NoiseElevReflectType)
  Radar_1_NoiseRange/1 -> Mux_Radar_1_TA/12(NoiseRange)
  Radar_1_NoiseRangeType/1 -> Mux_Radar_1_TA/13(NoiseRangeType)
  Mux_Radar_1_TA/1(TA) -> Radar_1_TA/1
  PointCloudSensor_1/1 -> PointCloudSensor_1_Range_Demux/1(In1), PointCloudSensor_1_Angles_Demux/1(In2), PointCloudSensor_1_Intensity_Demux/1(In1)
  PointCloudSensor_1_Location/1 -> Mux_PointCloudSensor_1_TA/1(Location)
  PointCloudSensor_1_Orientation/1 -> Mux_PointCloudSensor_1_TA/2(Orientation)
  PointCloudSensor_1_FovAzimuth/1 -> Mux_PointCloudSensor_1_TA/3(FovAzimuth)
  PointCloudSensor_1_FovElevation/1 -> Mux_PointCloudSensor_1_TA/4(FovElevation)
  Mux_PointCloudSensor_1_TA/1(TA) -> PointCloudSensor_1_TA/1
  PointCloudSensor_2/1 -> PointCloudSensor_2_Range_Demux/1(In1), PointCloudSensor_2_Angles_Demux/1(In2), PointCloudSensor_2_Intensity_Demux/1(In1)
  PointCloudSensor_2_Location/1 -> Mux_PointCloudSensor_2_TA/1(Location)
  PointCloudSensor_2_Orientation/1 -> Mux_PointCloudSensor_2_TA/2(Orientation)
  PointCloudSensor_2_FovAzimuth/1 -> Mux_PointCloudSensor_2_TA/3(FovAzimuth)
  PointCloudSensor_2_FovElevation/1 -> Mux_PointCloudSensor_2_TA/4(FovElevation)
  Mux_PointCloudSensor_2_TA/1(TA) -> PointCloudSensor_2_TA/1
  PointCloudSensor_3/1 -> PointCloudSensor_3_Range_Demux/1(In1), PointCloudSensor_3_Angles_Demux/1(In2), PointCloudSensor_3_Intensity_Demux/1(In1)
  PointCloudSensor_3_Location/1 -> Mux_PointCloudSensor_3_TA/1(Location)
  PointCloudSensor_3_Orientation/1 -> Mux_PointCloudSensor_3_TA/2(Orientation)
  PointCloudSensor_3_FovAzimuth/1 -> Mux_PointCloudSensor_3_TA/3(FovAzimuth)
  PointCloudSensor_3_FovElevation/1 -> Mux_PointCloudSensor_3_TA/4(FovElevation)
  Mux_PointCloudSensor_3_TA/1(TA) -> PointCloudSensor_3_TA/1
  PointCloudSensor_4/1 -> PointCloudSensor_4_Range_Demux/1(In1), PointCloudSensor_4_Angles_Demux/1(In2), PointCloudSensor_4_Intensity_Demux/1(In1)
  PointCloudSensor_4_Location/1 -> Mux_PointCloudSensor_4_TA/1(Location)
  PointCloudSensor_4_Orientation/1 -> Mux_PointCloudSensor_4_TA/2(Orientation)
  PointCloudSensor_4_FovAzimuth/1 -> Mux_PointCloudSensor_4_TA/3(FovAzimuth)
  PointCloudSensor_4_FovElevation/1 -> Mux_PointCloudSensor_4_TA/4(FovElevation)
  Mux_PointCloudSensor_4_TA/1(TA) -> PointCloudSensor_4_TA/1
  CameraSensor_2/1 -> CameraSensor_2_CM_Demux/1(In1)
  CameraSensor_2_CM_Demux/1(R) -> CameraSensor_2_CM_Display/1
  CameraSensor_2_CM_Demux/2(G) -> CameraSensor_2_CM_Display/2
  CameraSensor_2_CM_Demux/3(B) -> CameraSensor_2_CM_Display/3
  CameraSensor_2_Location/1 -> Mux_CameraSensor_2_TA/1(Location)
  CameraSensor_2_Orientation/1 -> Mux_CameraSensor_2_TA/2(Orientation)
  CameraSensor_2_IntensityFactorRGBMono/1 -> Mux_CameraSensor_2_TA/3(IntensityFactorRGBMono)
  CameraSensor_2_FoVAzimuth/1 -> Mux_CameraSensor_2_TA/4(FoVAzimuth)
  CameraSensor_2_FoVElevation/1 -> Mux_CameraSensor_2_TA/5(FoVElevation)
  CameraSensor_2_MisAlignMountPos/1 -> Mux_CameraSensor_2_TA/6(MisAlignMountPos)
  CameraSensor_2_MisAlignMountOrient/1 -> Mux_CameraSensor_2_TA/7(MisAlignMountOrient)
  Mux_CameraSensor_2_TA/1(TA) -> CameraSensor_2_TA/1
  HumViewCamera/1 -> HumViewCamera_CM_Demux/1(In1)
  HumViewCamera_CM_Demux/1(R) -> HumViewCamera_CM_Display/1
  HumViewCamera_CM_Demux/2(G) -> HumViewCamera_CM_Display/2
  HumViewCamera_CM_Demux/3(B) -> HumViewCamera_CM_Display/3
  HumViewCamera_Location/1 -> Mux_HumViewCamera_TA/1(Location)
  HumViewCamera_Orientation/1 -> Mux_HumViewCamera_TA/2(Orientation)
  HumViewCamera_IntensityFactorRGBMono/1 -> Mux_HumViewCamera_TA/3(IntensityFactorRGBMono)
  HumViewCamera_FoVAzimuth/1 -> Mux_HumViewCamera_TA/4(FoVAzimuth)
  HumViewCamera_FoVElevation/1 -> Mux_HumViewCamera_TA/5(FoVElevation)
  HumViewCamera_MisAlignMountPos/1 -> Mux_HumViewCamera_TA/6(MisAlignMountPos)
  HumViewCamera_MisAlignMountOrient/1 -> Mux_HumViewCamera_TA/7(MisAlignMountOrient)
  Mux_HumViewCamera_TA/1(TA) -> HumViewCamera_TA/1
  CameraSensor_4/1 -> CameraSensor_4_CM_Demux/1(In1)
  CameraSensor_4_CM_Demux/1(R) -> CameraSensor_4_CM_Display/1
  CameraSensor_4_CM_Demux/2(G) -> CameraSensor_4_CM_Display/2
  CameraSensor_4_CM_Demux/3(B) -> CameraSensor_4_CM_Display/3
  CameraSensor_4_Location/1 -> Mux_CameraSensor_4_TA/1(Location)
  CameraSensor_4_Orientation/1 -> Mux_CameraSensor_4_TA/2(Orientation)
  CameraSensor_4_IntensityFactorRGBMono/1 -> Mux_CameraSensor_4_TA/3(IntensityFactorRGBMono)
  CameraSensor_4_FoVAzimuth/1 -> Mux_CameraSensor_4_TA/4(FoVAzimuth)
  CameraSensor_4_FoVElevation/1 -> Mux_CameraSensor_4_TA/5(FoVElevation)
  CameraSensor_4_MisAlignMountPos/1 -> Mux_CameraSensor_4_TA/6(MisAlignMountPos)
  CameraSensor_4_MisAlignMountOrient/1 -> Mux_CameraSensor_4_TA/7(MisAlignMountOrient)
  Mux_CameraSensor_4_TA/1(TA) -> CameraSensor_4_TA/1
  CameraSensor_3/1 -> CameraSensor_3_CM_Demux/1(In1)
  CameraSensor_3_CM_Demux/1(R) -> CameraSensor_3_CM_Display/1
  CameraSensor_3_CM_Demux/2(G) -> CameraSensor_3_CM_Display/2
  CameraSensor_3_CM_Demux/3(B) -> CameraSensor_3_CM_Display/3
  CameraSensor_3_Location/1 -> Mux_CameraSensor_3_TA/1(Location)
  CameraSensor_3_Orientation/1 -> Mux_CameraSensor_3_TA/2(Orientation)
  CameraSensor_3_IntensityFactorRGBMono/1 -> Mux_CameraSensor_3_TA/3(IntensityFactorRGBMono)
  CameraSensor_3_FoVAzimuth/1 -> Mux_CameraSensor_3_TA/4(FoVAzimuth)
  CameraSensor_3_FoVElevation/1 -> Mux_CameraSensor_3_TA/5(FoVElevation)
  CameraSensor_3_MisAlignMountPos/1 -> Mux_CameraSensor_3_TA/6(MisAlignMountPos)
  CameraSensor_3_MisAlignMountOrient/1 -> Mux_CameraSensor_3_TA/7(MisAlignMountOrient)
  Mux_CameraSensor_3_TA/1(TA) -> CameraSensor_3_TA/1
  Camera_1/1 -> Camera_1_CM_Demux/1(In1)
  Camera_1_CM_Demux/1(R) -> Camera_1_CM_Display/1
  Camera_1_CM_Demux/2(G) -> Camera_1_CM_Display/2
  Camera_1_CM_Demux/3(B) -> Camera_1_CM_Display/3
  Camera_1_Location/1 -> Mux_Camera_1_TA/1(Location)
  Camera_1_Orientation/1 -> Mux_Camera_1_TA/2(Orientation)
  Camera_1_IntensityFactorRGBMono/1 -> Mux_Camera_1_TA/3(IntensityFactorRGBMono)
  Camera_1_FoVAzimuth/1 -> Mux_Camera_1_TA/4(FoVAzimuth)
  Camera_1_FoVElevation/1 -> Mux_Camera_1_TA/5(FoVElevation)
  Camera_1_MisAlignMountPos/1 -> Mux_Camera_1_TA/6(MisAlignMountPos)
  Camera_1_MisAlignMountOrient/1 -> Mux_Camera_1_TA/7(MisAlignMountOrient)
  Mux_Camera_1_TA/1(TA) -> Camera_1_TA/1
  Camera_tl/1 -> Camera_tl_CM_Demux/1(In1)
  Camera_tl_CM_Demux/1(R) -> Camera_tl_CM_Display/1
  Camera_tl_CM_Demux/2(G) -> Camera_tl_CM_Display/2
  Camera_tl_CM_Demux/3(B) -> Camera_tl_CM_Display/3
  Camera_tl_Location/1 -> Mux_Camera_tl_TA/1(Location)
  Camera_tl_Orientation/1 -> Mux_Camera_tl_TA/2(Orientation)
  Camera_tl_IntensityFactorRGBMono/1 -> Mux_Camera_tl_TA/3(IntensityFactorRGBMono)
  Camera_tl_FoVAzimuth/1 -> Mux_Camera_tl_TA/4(FoVAzimuth)
  Camera_tl_FoVElevation/1 -> Mux_Camera_tl_TA/5(FoVElevation)
  Camera_tl_MisAlignMountPos/1 -> Mux_Camera_tl_TA/6(MisAlignMountPos)
  Camera_tl_MisAlignMountOrient/1 -> Mux_Camera_tl_TA/7(MisAlignMountOrient)
  Mux_Camera_tl_TA/1(TA) -> Camera_tl_TA/1
  Camera_2/1 -> Camera_2_CM_Demux/1(In1)
  Camera_2_CM_Demux/1(R) -> Camera_2_CM_Display/1
  Camera_2_CM_Demux/2(G) -> Camera_2_CM_Display/2
  Camera_2_CM_Demux/3(B) -> Camera_2_CM_Display/3
  Camera_2_Location/1 -> Mux_Camera_2_TA/1(Location)
  Camera_2_Orientation/1 -> Mux_Camera_2_TA/2(Orientation)
  Camera_2_IntensityFactorRGBMono/1 -> Mux_Camera_2_TA/3(IntensityFactorRGBMono)
  Camera_2_FoVAzimuth/1 -> Mux_Camera_2_TA/4(FoVAzimuth)
  Camera_2_FoVElevation/1 -> Mux_Camera_2_TA/5(FoVElevation)
  Camera_2_MisAlignMountPos/1 -> Mux_Camera_2_TA/6(MisAlignMountPos)
  Camera_2_MisAlignMountOrient/1 -> Mux_Camera_2_TA/7(MisAlignMountOrient)
  Mux_Camera_2_TA/1(TA) -> Camera_2_TA/1
  Dynamics_Empty/1(State) -> STATE_BMW_X5_SUV_1_rc/1
  PointCloudSensor_1_Angles_Demux/1(Theta) -> Terminator_1/1
  PointCloudSensor_1_Angles_Demux/2(Phi) -> Terminator_2/1
  PointCloudSensor_1_Intensity_Demux/1(Intensity) -> Terminator_3/1
  PointCloudSensor_1_Range_Demux/1(Range) -> Terminator_4/1
  PointCloudSensor_2_Angles_Demux/1(Theta) -> Terminator_5/1
  PointCloudSensor_2_Angles_Demux/2(Phi) -> Terminator_6/1
  PointCloudSensor_2_Intensity_Demux/1(Intensity) -> Terminator_7/1
  PointCloudSensor_2_Range_Demux/1(Range) -> Terminator_8/1
  PointCloudSensor_3_Angles_Demux/1(Theta) -> Terminator_9/1
  PointCloudSensor_3_Angles_Demux/2(Phi) -> Terminator_10/1
  PointCloudSensor_3_Intensity_Demux/1(Intensity) -> Terminator_11/1
  PointCloudSensor_3_Range_Demux/1(Range) -> Terminator_12/1
  PointCloudSensor_4_Angles_Demux/1(Theta) -> Terminator_13/1
  PointCloudSensor_4_Angles_Demux/2(Phi) -> Terminator_14/1
  PointCloudSensor_4_Intensity_Demux/1(Intensity) -> Terminator_15/1
  PointCloudSensor_4_Range_Demux/1(Range) -> Terminator_16/1
  Radar_1_Demux/1(Radar Data) -> Terminator_17/1
  SELF_Demux/1(x [m]) -> Terminator_18/1
  SELF_Demux/2(y [m]) -> Terminator_19/1
  SELF_Demux/3(z [m]) -> Terminator_20/1
  SELF_Demux/4(rotx [deg]) -> Terminator_21/1
  SELF_Demux/5(roty [deg]) -> Terminator_22/1
  SELF_Demux/6(rotz [deg]) -> Terminator_23/1
  SELF_Demux/7(GPS lat [deg]) -> Terminator_24/1
  SELF_Demux/8(GPS long [deg]) -> Terminator_25/1
  SELF_Demux/9(GPS alt [m]) -> Terminator_26/1
  SELF_Demux/10(velocity [m/s]) -> Terminator_27/1
  SELF_Demux/11(heading [deg]) -> Terminator_28/1
  SELF_Demux/12(yaw rate [deg/s]) -> Terminator_29/1

== system Open_scen_lucie_test_cs/CameraSensor_2 ==
  Sensor : S-Function  FunctionName=sfun_Camera  Parameters=sensorID, dataWidth, dataHeight, channelsPerImage, numberOfImages, timestep  SFunctionDeploymentMode=off  EnableBusSupport=off  mask(PreScan Source Block: Camera Sensor){sensorID=411, dataWidth=720, dataHeight=2880, channelsPerImage=3, numberOfImages=1, timestep=1/20}
      mask prompts: sensorID "Sensor ID"; dataWidth "Data width"; dataHeight "Data Height"; channelsPerImage "Channels per image"; numberOfImages "Number of images"; timestep "MATLAB timestep:"
      mask help: The Camera Sensor provides a color or monochrome image.
      mask Help: eval('openHelp(457)')
      mask Display: image(imread('CameraSensor.png'))
  CameraSensor_2 : Outport  Tag=outport/Camera/CameraSensor  OutDataTypeStr=uint8  SampleTime=1/20
  wires:
  Sensor/1 -> CameraSensor_2/1

== system Open_scen_lucie_test_cs/CameraSensor_2_TA ==
  CameraSensor_2_TA : Inport  Tag=inport/Camera_TA/CameraSensor  OutDataTypeStr=Bus: PRESCAN_CAMERASENSOR_TA  PortDimensions=1  SampleTime=1/60  BusOutputAsStruct=on
  Actuator : S-Function  FunctionName=sfun_Camera_TA  Parameters=sensorID, timestep  SFunctionDeploymentMode=off  EnableBusSupport=off  mask(Camera Sensor Test Automation){sensorID=411, timestep=1/60}
      mask prompts: sensorID "Sensor ID"; timestep "MATLAB timestep:"
      mask help:
      | The TA Sink block updates the Test Automation variables in the Simulation.
      |
      | Note: All angles are expressed in degrees
      |
      | Remarks:
      | TIS: Drift Type:
      |   0: None
      |   1: Gaussian
      |   2: Unidirectional
      |
      | TIS: Noise Type:
      |   0: Additive
      |   1: Multiplicative
      |
      | AIR: Detection Type:
      |   0: BoundingBox
      |   1: Bounding Box Center
      |   2: CenterOfGravity
      |
      | Antenna Tx: Range
      |   -1: Infinite
      |
      | For more information, please click Help.
      mask Help: eval('openHelp(633)')
      mask Display: image(imread('TA.png'))
  wires:
  CameraSensor_2_TA/1 -> Actuator/1
